simulink model "randdsb"  (R2015a)
settings: Solver=ode45  StartTime=0.0  StopTime=inf  RelTol=1e-3
libraries: commanapbnd3 x2, commchan3 x1, dspsrcs4 x1
settings Model: Creator=Saurabh Roy  LastModifiedBy=Saurabh Roy

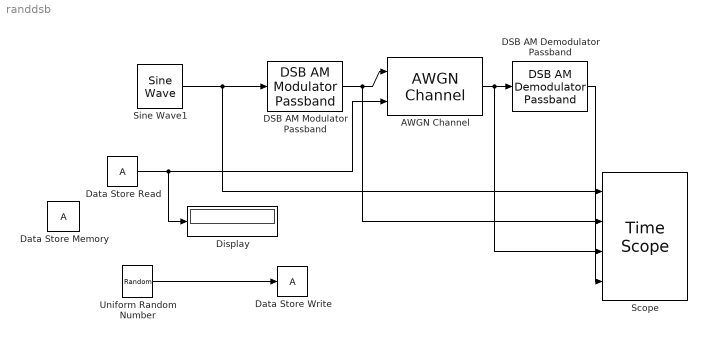
== system randdsb ==
  AWGN Channel : commchan3/AWGN Channel  InputProcessing=Columns as channels (frame based)  seed=67  noiseMode=Variance from port  EbNodB=25  EsNodB=10  SNRdB=10  bitsPerSym=1  Ps=1  Tsym=1  variance=1
  DSB AM Demodulator Passband : commanapbnd3/DSB AM Demodulator Passband  Fc=300  Ph=0  method=Butterworth  n=4  cf=300  Rp=0.1  Rs=50  Offset=1
  DSB AM Modulator Passband : commanapbnd3/DSB AM Modulator Passband  Fc=300  Ph=0  Offset=1
  Data Store Memory : DataStoreMemory  ReadBeforeWriteMsg=warning  WriteAfterWriteMsg=warning  WriteAfterReadMsg=warning
  Data Store Read : DataStoreRead
  Data Store Write : DataStoreWrite
  Display : Display
  Scope : TimeScope  NumInputPorts=4
  Sine Wave1 : dspsrcs4/Sine Wave  Amplitude=5  Frequency=0.01  Phase=0  SampleMode=Discrete  OutComplex=Real  CompMethod=Trigonometric fcn  TableSize=Speed  SampleTime=1/1000  SamplesPerFrame=1  ResetState=Restart at time zero  dataType=double  wordLen=16  udDataType=sfix(16)  fracBitsMode=Best precision  numFracBits=15  OutDataTypeStr=double  LastOutDataTypeStr=double
  Uniform Random Number : UniformRandomNumber  Minimum=0  Maximum=10  SampleTime=0.1
  wires:
  Sine Wave1/1 -> Scope/1, DSB AM Modulator Passband/1
  AWGN Channel/1 -> Scope/3, DSB AM Demodulator Passband/1
  DSB AM Modulator Passband/1 -> Scope/2, AWGN Channel/1
  DSB AM Demodulator Passband/1 -> Scope/4
  Uniform Random Number/1 -> Data Store Write/1
  Data Store Read/1 -> Display/1, AWGN Channel/2
